simulink model "SIFT_final"  (R2015a)
settings: Solver=ode45  StartTime=0.0  StopTime=10.0  RelTol=1e-3
InitFcn:
  | %% DSPBuilder Start
  | alt_dspbuilder_update_model(bdroot)
  | %% DSPBuilder End
libraries: allblocks_alteradspbuilder2 x1826
(part 2 of 24)

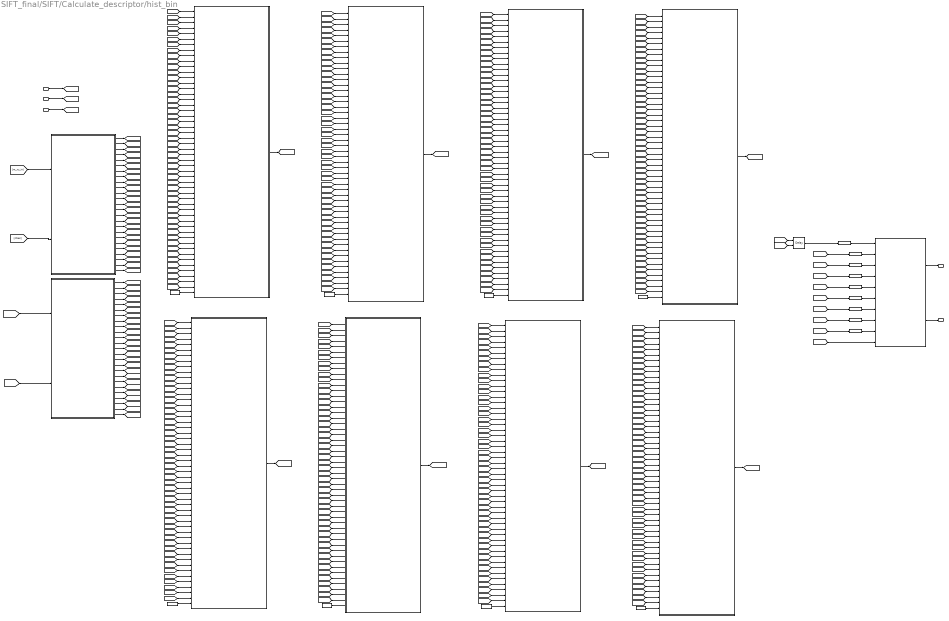
== system SIFT_final/SIFT/Calculate_descriptor/hist_bin ==
  m_xy_In : Inport
  orien_In : Inport  Port=2
  clken : Inport  Port=3
  AltBus : allblocks_alteradspbuilder2/AltBus  BusType=Unsigned Integer  bwl=16  bwr=0  saturate=off  floatingPointInput=on  floatingPointOutput=on  logOutputs=off  logFile=C:\Users\ASUS\Desktop\final_sift_fpga\tb_SIFT_final\SIFT%5Ffinal_SIFT_Calculate%5Fdescriptor_hist%5Fbin_AltBus.fixedpointlog
  AltBus1 : allblocks_alteradspbuilder2/AltBus  BusType=Unsigned Integer  bwl=16  bwr=0  saturate=off  floatingPointInput=on  floatingPointOutput=on  logOutputs=off  logFile=C:\Users\ASUS\Desktop\final_sift_fpga\tb_SIFT_final\SIFT%5Ffinal_SIFT_Calculate%5Fdescriptor_hist%5Fbin_AltBus1.fixedpointlog
  AltBus2 : allblocks_alteradspbuilder2/AltBus  BusType=Unsigned Integer  bwl=16  bwr=0  saturate=off  floatingPointInput=on  floatingPointOutput=on  logOutputs=off  logFile=C:\Users\ASUS\Desktop\final_sift_fpga\tb_SIFT_final\SIFT%5Ffinal_SIFT_Calculate%5Fdescriptor_hist%5Fbin_AltBus2.fixedpointlog
  AltBus3 : allblocks_alteradspbuilder2/AltBus  BusType=Unsigned Integer  bwl=16  bwr=0  saturate=off  floatingPointInput=on  floatingPointOutput=on  logOutputs=off  logFile=C:\Users\ASUS\Desktop\final_sift_fpga\tb_SIFT_final\SIFT%5Ffinal_SIFT_Calculate%5Fdescriptor_hist%5Fbin_AltBus3.fixedpointlog
  AltBus4 : allblocks_alteradspbuilder2/AltBus  BusType=Unsigned Integer  bwl=16  bwr=0  saturate=off  floatingPointInput=on  floatingPointOutput=on  logOutputs=off  logFile=C:\Users\ASUS\Desktop\final_sift_fpga\tb_SIFT_final\SIFT%5Ffinal_SIFT_Calculate%5Fdescriptor_hist%5Fbin_AltBus4.fixedpointlog
  AltBus5 : allblocks_alteradspbuilder2/AltBus  BusType=Unsigned Integer  bwl=16  bwr=0  saturate=off  floatingPointInput=on  floatingPointOutput=on  logOutputs=off  logFile=C:\Users\ASUS\Desktop\final_sift_fpga\tb_SIFT_final\SIFT%5Ffinal_SIFT_Calculate%5Fdescriptor_hist%5Fbin_AltBus5.fixedpointlog
  AltBus6 : allblocks_alteradspbuilder2/AltBus  BusType=Unsigned Integer  bwl=16  bwr=0  saturate=off  floatingPointInput=on  floatingPointOutput=on  logOutputs=off  logFile=C:\Users\ASUS\Desktop\final_sift_fpga\tb_SIFT_final\SIFT%5Ffinal_SIFT_Calculate%5Fdescriptor_hist%5Fbin_AltBus6.fixedpointlog
  AltBus7 : allblocks_alteradspbuilder2/AltBus  BusType=Unsigned Integer  bwl=16  bwr=0  saturate=off  floatingPointInput=on  floatingPointOutput=on  logOutputs=off  logFile=C:\Users\ASUS\Desktop\final_sift_fpga\tb_SIFT_final\SIFT%5Ffinal_SIFT_Calculate%5Fdescriptor_hist%5Fbin_AltBus7.fixedpointlog
  AltBus8 : allblocks_alteradspbuilder2/AltBus  BusType=Unsigned Integer  bwl=3  bwr=0  saturate=off  floatingPointInput=on  floatingPointOutput=on  logOutputs=off  logFile=C:\Users\ASUS\Desktop\final_sift_fpga\tb_SIFT_final\SIFT%5Ffinal_SIFT_Calculate%5Fdescriptor_hist%5Fbin_AltBus8.fixedpointlog
  Bus_Concatenation : Subsystem
  Constant : allblocks_alteradspbuilder2/Constant  mask_cst=0  BusType=Unsigned Integer  bwl=8  bwr=0  roundMode=Truncate  satMode=Wrap  SpecifyClock=off  allowFloatingPointOverride=on  logOutputs=off  logFile=C:\Users\ASUS\Desktop\final_sift_fpga\tb_SIFT_final\SIFT%5Ffinal_SIFT_Calculate%5Fdescriptor_hist%5Fbin_Constant.fixedpointlog
  Constant1 : allblocks_alteradspbuilder2/Constant  mask_cst=1  BusType=Unsigned Integer  bwl=8  bwr=0  roundMode=Truncate  satMode=Wrap  SpecifyClock=off  allowFloatingPointOverride=on  logOutputs=off  logFile=C:\Users\ASUS\Desktop\final_sift_fpga\tb_SIFT_final\SIFT%5Ffinal_SIFT_Calculate%5Fdescriptor_hist%5Fbin_Constant1.fixedpointlog
  Constant2 : allblocks_alteradspbuilder2/Constant  mask_cst=2  BusType=Unsigned Integer  bwl=8  bwr=0  roundMode=Truncate  satMode=Wrap  SpecifyClock=off  allowFloatingPointOverride=on  logOutputs=off  logFile=C:\Users\ASUS\Desktop\final_sift_fpga\tb_SIFT_final\SIFT%5Ffinal_SIFT_Calculate%5Fdescriptor_hist%5Fbin_Constant2.fixedpointlog
  Constant3 : allblocks_alteradspbuilder2/Constant  mask_cst=3  BusType=Unsigned Integer  bwl=8  bwr=0  roundMode=Truncate  satMode=Wrap  SpecifyClock=off  allowFloatingPointOverride=on  logOutputs=off  logFile=C:\Users\ASUS\Desktop\final_sift_fpga\tb_SIFT_final\SIFT%5Ffinal_SIFT_Calculate%5Fdescriptor_hist%5Fbin_Constant3.fixedpointlog
  Constant4 : allblocks_alteradspbuilder2/Constant  mask_cst=4  BusType=Unsigned Integer  bwl=8  bwr=0  roundMode=Truncate  satMode=Wrap  SpecifyClock=off  allowFloatingPointOverride=on  logOutputs=off  logFile=C:\Users\ASUS\Desktop\final_sift_fpga\tb_SIFT_final\SIFT%5Ffinal_SIFT_Calculate%5Fdescriptor_hist%5Fbin_Constant4.fixedpointlog
  Constant5 : allblocks_alteradspbuilder2/Constant  mask_cst=5  BusType=Unsigned Integer  bwl=8  bwr=0  roundMode=Truncate  satMode=Wrap  SpecifyClock=off  allowFloatingPointOverride=on  logOutputs=off  logFile=C:\Users\ASUS\Desktop\final_sift_fpga\tb_SIFT_final\SIFT%5Ffinal_SIFT_Calculate%5Fdescriptor_hist%5Fbin_Constant5.fixedpointlog
  Constant6 : allblocks_alteradspbuilder2/Constant  mask_cst=6  BusType=Unsigned Integer  bwl=8  bwr=0  roundMode=Truncate  satMode=Wrap  SpecifyClock=off  allowFloatingPointOverride=on  logOutputs=off  logFile=C:\Users\ASUS\Desktop\final_sift_fpga\tb_SIFT_final\SIFT%5Ffinal_SIFT_Calculate%5Fdescriptor_hist%5Fbin_Constant6.fixedpointlog
  Constant7 : allblocks_alteradspbuilder2/Constant  mask_cst=7  BusType=Unsigned Integer  bwl=8  bwr=0  roundMode=Truncate  satMode=Wrap  SpecifyClock=off  allowFloatingPointOverride=on  logOutputs=off  logFile=C:\Users\ASUS\Desktop\final_sift_fpga\tb_SIFT_final\SIFT%5Ffinal_SIFT_Calculate%5Fdescriptor_hist%5Fbin_Constant7.fixedpointlog
  Delay : allblocks_alteradspbuilder2/Delay  pipeline=5+16  pipeline_display=21  ClockPhase=1  use_ena=on  use_sclr=off  allowFloatingPointOverride=on  logOutputs=off  logFile=C:\Users\ASUS\Desktop\final_sift_fpga\tb_SIFT_final\SIFT%5Ffinal_SIFT_Calculate%5Fdescriptor_hist%5Fbin_Delay.fixedpointlog  use_init=off  reset_value=1
  Line_buffer_5x5 : Subsystem
  Line_buffer_5x5_1 : Subsystem
  hist_bin1 : Subsystem
  hist_bin2 : Subsystem
  hist_bin3 : Subsystem
  hist_bin4 : Subsystem
  hist_bin5 : Subsystem
  hist_bin6 : Subsystem
  hist_bin7 : Subsystem
  hist_bin8 : Subsystem
  hist_bin_out : Outport
  Orien_out : Outport  Port=2
  wires:
  [m_xy_in] -> Line_buffer_5x5/1(dataIn)
  [clken] -> Line_buffer_5x5/2(clken)
  [clken] -> Line_buffer_5x5_1/2(clken)
  [orien_in] -> Line_buffer_5x5_1/1(dataIn)
  clken/1 -> [clken]
  Line_buffer_5x5_1/21(Out40) -> [orien_40]
  Line_buffer_5x5_1/19(Out33) -> [orien_33]
  Line_buffer_5x5_1/8(Out12) -> [orien_12]
  Line_buffer_5x5_1/14(Out23) -> [orien_23]
  Line_buffer_5x5_1/18(Out32) -> [orien_32]
  Line_buffer_5x5_1/20(Out34) -> [orien_34]
  Line_buffer_5x5_1/2(Out01) -> [orien_01]
  Line_buffer_5x5_1/7(Out11) -> [orien_11]
  Line_buffer_5x5_1/11(Out20) -> [orien_20]
  Line_buffer_5x5_1/13(Out22) -> [orien_22]
  Line_buffer_5x5_1/17(Out31) -> [orien_31]
  Line_buffer_5x5_1/25(Out44) -> [orien_44]
  Line_buffer_5x5_1/3(Out02) -> [orien_02]
  Line_buffer_5x5_1/5(Out04) -> [orien_04]
  Line_buffer_5x5_1/23(Out42) -> [orien_42]
  Line_buffer_5x5_1/24(Out43) -> [orien_43]
  Line_buffer_5x5_1/6(Out10) -> [orien_10]
  Line_buffer_5x5_1/1(Out00) -> [orien_00]
  Line_buffer_5x5_1/22(Out41) -> [orien_41]
  Line_buffer_5x5_1/15(Out24) -> [orien_24]
  Line_buffer_5x5_1/4(Out03) -> [orien_03]
  Line_buffer_5x5_1/9(Out13) -> [orien_13]
  Line_buffer_5x5_1/10(Out14) -> [orien_14]
  Line_buffer_5x5_1/12(Out21) -> [orien_21]
  Line_buffer_5x5_1/16(Out30) -> [orien_30]
  Line_buffer_5x5/24(Out43) -> [m_xy_43]
  Line_buffer_5x5/21(Out40) -> [m_xy_40]
  Line_buffer_5x5/23(Out42) -> [m_xy_42]
  Line_buffer_5x5/22(Out41) -> [m_xy_41]
  Line_buffer_5x5/25(Out44) -> [m_xy_44]
  Line_buffer_5x5/12(Out21) -> [m_xy_21]
  Line_buffer_5x5/15(Out24) -> [m_xy_24]
  Line_buffer_5x5/19(Out33) -> [m_xy_33]
  Line_buffer_5x5/18(Out32) -> [m_xy_32]
  Line_buffer_5x5/13(Out22) -> [m_xy_22]
  Line_buffer_5x5/11(Out20) -> [m_xy_20]
  Line_buffer_5x5/16(Out30) -> [m_xy_30]
  Line_buffer_5x5/14(Out23) -> [m_xy_23]
  Line_buffer_5x5/17(Out31) -> [m_xy_31]
  Line_buffer_5x5/20(Out34) -> [m_xy_34]
  Line_buffer_5x5/1(Out00) -> [m_xy_00]
  [m_xy_04] -> hist_bin1/5(Mxy_In04)
  Line_buffer_5x5/2(Out01) -> [m_xy_01]
  hist_bin1/1(bin_out) -> [hist_bin1]
  [m_xy_10] -> hist_bin1/6(Mxy_In10)
  Line_buffer_5x5/9(Out13) -> [m_xy_13]
  [m_xy_13] -> hist_bin1/9(Mxy_In13)
  Line_buffer_5x5/10(Out14) -> [m_xy_14]
  Line_buffer_5x5/6(Out10) -> [m_xy_10]
  Line_buffer_5x5/7(Out11) -> [m_xy_11]
  [m_xy_11] -> hist_bin1/7(Mxy_In11)
  [m_xy_12] -> hist_bin1/8(Mxy_In12)
  Line_buffer_5x5/8(Out12) -> [m_xy_12]
  [m_xy_14] -> hist_bin1/10(Mxy_In14)
  [m_xy_22] -> hist_bin1/13(Mxy_In22)
  [m_xy_40] -> hist_bin1/21(Mxy_In40)
  [m_xy_43] -> hist_bin1/24(Mxy_In43)
  [m_xy_42] -> hist_bin1/23(Mxy_In42)
  [m_xy_44] -> hist_bin1/25(Mxy_In44)
  [m_xy_24] -> hist_bin1/15(Mxy_In24)
  [m_xy_21] -> hist_bin1/12(Mxy_In21)
  [m_xy_20] -> hist_bin1/11(Mxy_In20)
  [m_xy_23] -> hist_bin1/14(Mxy_In23)
  [m_xy_41] -> hist_bin1/22(Mxy_In41)
  [m_xy_01] -> hist_bin1/2(Mxy_In01)
  Line_buffer_5x5/4(Out03) -> [m_xy_03]
  Line_buffer_5x5/5(Out04) -> [m_xy_04]
  Line_buffer_5x5/3(Out02) -> [m_xy_02]
  [m_xy_31] -> hist_bin1/17(Mxy_In31)
  [m_xy_30] -> hist_bin1/16(Mxy_In30)
  [m_xy_34] -> hist_bin1/20(Mxy_In34)
  [m_xy_33] -> hist_bin1/19(Mxy_In33)
  [m_xy_32] -> hist_bin1/18(Mxy_In32)
  [m_xy_03] -> hist_bin1/4(Mxy_In03)
  [m_xy_02] -> hist_bin1/3(Mxy_In02)
  [orien_10] -> hist_bin1/31(Orien_In10)
  [orien_42] -> hist_bin1/48(Orien_In42)
  [orien_01] -> hist_bin1/27(Orien_In01)
  [orien_20] -> hist_bin1/36(Orien_In20)
  [orien_31] -> hist_bin1/42(Orien_In31)
  [orien_33] -> hist_bin1/44(Orien_In33)
  [orien_21] -> hist_bin1/37(Orien_In21)
  [orien_24] -> hist_bin1/40(Orien_In24)
  [orien_03] -> hist_bin1/29(Orien_In03)
  [orien_30] -> hist_bin1/41(Orien_In30)
  [orien_12] -> hist_bin1/33(Orien_In12)
  [orien_23] -> hist_bin1/39(Orien_In23)
  [orien_32] -> hist_bin1/43(Orien_In32)
  [orien_41] -> hist_bin1/47(Orien_In41)
  [orien_43] -> hist_bin1/49(Orien_In43)
  [orien_02] -> hist_bin1/28(Orien_In02)
  [orien_00] -> hist_bin1/26(Orien_In00)
  [orien_11] -> hist_bin1/32(Orien_In11)
  [orien_34] -> hist_bin1/45(Orien_In34)
  [orien_22] -> hist_bin1/38(Orien_In22)
  [orien_04] -> hist_bin1/30(Orien_In04)
  [orien_14] -> hist_bin1/35(Orien_In14)
  [orien_44] -> hist_bin1/50(Orien_In44)
  [orien_13] -> hist_bin1/34(Orien_In13)
  [orien_40] -> hist_bin1/46(Orien_In40)
  [clken] -> hist_bin1/51(clken)
  Constant/1 -> hist_bin1/52(bin_in)
  [m_xy_02] -> hist_bin2/3(Mxy_In02)
  [m_xy_04] -> hist_bin2/5(Mxy_In04)
  [m_xy_10] -> hist_bin2/6(Mxy_In10)
  [m_xy_23] -> hist_bin2/14(Mxy_In23)
  [m_xy_31] -> hist_bin2/17(Mxy_In31)
  [m_xy_30] -> hist_bin2/16(Mxy_In30)
  [m_xy_12] -> hist_bin2/8(Mxy_In12)
  [m_xy_32] -> hist_bin2/18(Mxy_In32)
  [m_xy_13] -> hist_bin2/9(Mxy_In13)
  [m_xy_33] -> hist_bin2/19(Mxy_In33)
  [m_xy_41] -> hist_bin2/22(Mxy_In41)
  [m_xy_01] -> hist_bin2/2(Mxy_In01)
  [m_xy_14] -> hist_bin2/10(Mxy_In14)
  [m_xy_40] -> hist_bin2/21(Mxy_In40)
  [m_xy_43] -> hist_bin2/24(Mxy_In43)
  [m_xy_20] -> hist_bin2/11(Mxy_In20)
  [m_xy_22] -> hist_bin2/13(Mxy_In22)
  [m_xy_24] -> hist_bin2/15(Mxy_In24)
  [m_xy_34] -> hist_bin2/20(Mxy_In34)
  [m_xy_03] -> hist_bin2/4(Mxy_In03)
  [m_xy_00] -> hist_bin2/1(Mxy_In00)
  [m_xy_11] -> hist_bin2/7(Mxy_In11)
  [m_xy_21] -> hist_bin2/12(Mxy_In21)
  [orien_31] -> hist_bin2/42(Orien_In31)
  [orien_34] -> hist_bin2/45(Orien_In34)
  [m_xy_42] -> hist_bin2/23(Mxy_In42)
  [orien_01] -> hist_bin2/27(Orien_In01)
  [orien_00] -> hist_bin2/26(Orien_In00)
  [orien_04] -> hist_bin2/30(Orien_In04)
  [orien_13] -> hist_bin2/34(Orien_In13)
  [orien_20] -> hist_bin2/36(Orien_In20)
  [orien_24] -> hist_bin2/40(Orien_In24)
  [orien_33] -> hist_bin2/44(Orien_In33)
  [orien_32] -> hist_bin2/43(Orien_In32)
  [orien_41] -> hist_bin2/47(Orien_In41)
  [orien_11] -> hist_bin2/32(Orien_In11)
  [orien_21] -> hist_bin2/37(Orien_In21)
  [orien_14] -> hist_bin2/35(Orien_In14)
  [orien_22] -> hist_bin2/38(Orien_In22)
  [orien_23] -> hist_bin2/39(Orien_In23)
  [orien_02] -> hist_bin2/28(Orien_In02)
  [orien_10] -> hist_bin2/31(Orien_In10)
  [orien_12] -> hist_bin2/33(Orien_In12)
  [orien_30] -> hist_bin2/41(Orien_In30)
  [m_xy_44] -> hist_bin2/25(Mxy_In44)
  [orien_03] -> hist_bin2/29(Orien_In03)
  [orien_40] -> hist_bin2/46(Orien_In40)
  [clken] -> hist_bin2/51(clken)
  hist_bin2/1(bin_out) -> [hist_bin2]
  [orien_42] -> hist_bin2/48(Orien_In42)
  [orien_44] -> hist_bin2/50(Orien_In44)
  [orien_43] -> hist_bin2/49(Orien_In43)
  Constant1/1 -> hist_bin2/52(bin_in)
  [m_xy_00] -> hist_bin1/1(Mxy_In00)
  orien_In/1 -> [orien_in]
  m_xy_In/1 -> [m_xy_in]
  [m_xy_04] -> hist_bin3/5(Mxy_In04)
  hist_bin3/1(bin_out) -> [hist_bin3]
  [m_xy_10] -> hist_bin3/6(Mxy_In10)
  [m_xy_13] -> hist_bin3/9(Mxy_In13)
  [m_xy_11] -> hist_bin3/7(Mxy_In11)
  [m_xy_12] -> hist_bin3/8(Mxy_In12)
  [m_xy_14] -> hist_bin3/10(Mxy_In14)
  [m_xy_22] -> hist_bin3/13(Mxy_In22)
  [m_xy_40] -> hist_bin3/21(Mxy_In40)
  [m_xy_43] -> hist_bin3/24(Mxy_In43)
  [m_xy_42] -> hist_bin3/23(Mxy_In42)
  [m_xy_44] -> hist_bin3/25(Mxy_In44)
  [m_xy_24] -> hist_bin3/15(Mxy_In24)
  [m_xy_21] -> hist_bin3/12(Mxy_In21)
  [m_xy_20] -> hist_bin3/11(Mxy_In20)
  [m_xy_23] -> hist_bin3/14(Mxy_In23)
  [m_xy_41] -> hist_bin3/22(Mxy_In41)
  [m_xy_01] -> hist_bin3/2(Mxy_In01)
  [m_xy_31] -> hist_bin3/17(Mxy_In31)
  [m_xy_30] -> hist_bin3/16(Mxy_In30)
  [m_xy_34] -> hist_bin3/20(Mxy_In34)
  [m_xy_33] -> hist_bin3/19(Mxy_In33)
  [m_xy_32] -> hist_bin3/18(Mxy_In32)
  [m_xy_03] -> hist_bin3/4(Mxy_In03)
  [m_xy_02] -> hist_bin3/3(Mxy_In02)
  [orien_10] -> hist_bin3/31(Orien_In10)
  [orien_42] -> hist_bin3/48(Orien_In42)
  [orien_01] -> hist_bin3/27(Orien_In01)
  [orien_20] -> hist_bin3/36(Orien_In20)
  [orien_31] -> hist_bin3/42(Orien_In31)
  [orien_33] -> hist_bin3/44(Orien_In33)
  [orien_21] -> hist_bin3/37(Orien_In21)
  [orien_24] -> hist_bin3/40(Orien_In24)
  [orien_03] -> hist_bin3/29(Orien_In03)
  [orien_30] -> hist_bin3/41(Orien_In30)
  [orien_12] -> hist_bin3/33(Orien_In12)
  [orien_23] -> hist_bin3/39(Orien_In23)
  [orien_32] -> hist_bin3/43(Orien_In32)
  [orien_41] -> hist_bin3/47(Orien_In41)
  [orien_43] -> hist_bin3/49(Orien_In43)
  [orien_02] -> hist_bin3/28(Orien_In02)
  [orien_00] -> hist_bin3/26(Orien_In00)
  [orien_11] -> hist_bin3/32(Orien_In11)
  [orien_34] -> hist_bin3/45(Orien_In34)
  [orien_22] -> hist_bin3/38(Orien_In22)
  [orien_04] -> hist_bin3/30(Orien_In04)
  [orien_14] -> hist_bin3/35(Orien_In14)
  [orien_44] -> hist_bin3/50(Orien_In44)
  [orien_13] -> hist_bin3/34(Orien_In13)
  [orien_40] -> hist_bin3/46(Orien_In40)
  [clken] -> hist_bin3/51(clken)
  Constant2/1 -> hist_bin3/52(bin_in)
  [m_xy_02] -> hist_bin4/3(Mxy_In02)
  [m_xy_04] -> hist_bin4/5(Mxy_In04)
  [m_xy_10] -> hist_bin4/6(Mxy_In10)
  [m_xy_23] -> hist_bin4/14(Mxy_In23)
  [m_xy_31] -> hist_bin4/17(Mxy_In31)
  [m_xy_30] -> hist_bin4/16(Mxy_In30)
  [m_xy_12] -> hist_bin4/8(Mxy_In12)
  [m_xy_32] -> hist_bin4/18(Mxy_In32)
  [m_xy_13] -> hist_bin4/9(Mxy_In13)
  [m_xy_33] -> hist_bin4/19(Mxy_In33)
  [m_xy_41] -> hist_bin4/22(Mxy_In41)
  [m_xy_01] -> hist_bin4/2(Mxy_In01)
  [m_xy_14] -> hist_bin4/10(Mxy_In14)
  [m_xy_40] -> hist_bin4/21(Mxy_In40)
  [m_xy_43] -> hist_bin4/24(Mxy_In43)
  [m_xy_20] -> hist_bin4/11(Mxy_In20)
  [m_xy_22] -> hist_bin4/13(Mxy_In22)
  [m_xy_24] -> hist_bin4/15(Mxy_In24)
  [m_xy_34] -> hist_bin4/20(Mxy_In34)
  [m_xy_03] -> hist_bin4/4(Mxy_In03)
  [m_xy_00] -> hist_bin4/1(Mxy_In00)
  [m_xy_11] -> hist_bin4/7(Mxy_In11)
  [m_xy_21] -> hist_bin4/12(Mxy_In21)
  [orien_31] -> hist_bin4/42(Orien_In31)
  [orien_34] -> hist_bin4/45(Orien_In34)
  [m_xy_42] -> hist_bin4/23(Mxy_In42)
  [orien_01] -> hist_bin4/27(Orien_In01)
  [orien_00] -> hist_bin4/26(Orien_In00)
  [orien_04] -> hist_bin4/30(Orien_In04)
  [orien_13] -> hist_bin4/34(Orien_In13)
  [orien_20] -> hist_bin4/36(Orien_In20)
  [orien_24] -> hist_bin4/40(Orien_In24)
  [orien_33] -> hist_bin4/44(Orien_In33)
  [orien_32] -> hist_bin4/43(Orien_In32)
  [orien_41] -> hist_bin4/47(Orien_In41)
  [orien_11] -> hist_bin4/32(Orien_In11)
  [orien_21] -> hist_bin4/37(Orien_In21)
  [orien_14] -> hist_bin4/35(Orien_In14)
  [orien_22] -> hist_bin4/38(Orien_In22)
  [orien_23] -> hist_bin4/39(Orien_In23)
  [orien_02] -> hist_bin4/28(Orien_In02)
  [orien_10] -> hist_bin4/31(Orien_In10)
  [orien_12] -> hist_bin4/33(Orien_In12)
  [orien_30] -> hist_bin4/41(Orien_In30)
  [m_xy_44] -> hist_bin4/25(Mxy_In44)
  [orien_03] -> hist_bin4/29(Orien_In03)
  [orien_40] -> hist_bin4/46(Orien_In40)
  [clken] -> hist_bin4/51(clken)
  hist_bin4/1(bin_out) -> [hist_bin4]
  [orien_42] -> hist_bin4/48(Orien_In42)
  [orien_44] -> hist_bin4/50(Orien_In44)
  [orien_43] -> hist_bin4/49(Orien_In43)
  Constant3/1 -> hist_bin4/52(bin_in)
  [m_xy_00] -> hist_bin3/1(Mxy_In00)
  [m_xy_04] -> hist_bin5/5(Mxy_In04)
  hist_bin5/1(bin_out) -> [hist_bin5]
  [m_xy_10] -> hist_bin5/6(Mxy_In10)
  [m_xy_13] -> hist_bin5/9(Mxy_In13)
  [m_xy_11] -> hist_bin5/7(Mxy_In11)
  [m_xy_12] -> hist_bin5/8(Mxy_In12)
  [m_xy_14] -> hist_bin5/10(Mxy_In14)
  [m_xy_22] -> hist_bin5/13(Mxy_In22)
  [m_xy_40] -> hist_bin5/21(Mxy_In40)
  [m_xy_43] -> hist_bin5/24(Mxy_In43)
  [m_xy_42] -> hist_bin5/23(Mxy_In42)
  [m_xy_44] -> hist_bin5/25(Mxy_In44)
  [m_xy_24] -> hist_bin5/15(Mxy_In24)
  [m_xy_21] -> hist_bin5/12(Mxy_In21)
  [m_xy_20] -> hist_bin5/11(Mxy_In20)
  [m_xy_23] -> hist_bin5/14(Mxy_In23)
  [m_xy_41] -> hist_bin5/22(Mxy_In41)
  [m_xy_01] -> hist_bin5/2(Mxy_In01)
  [m_xy_31] -> hist_bin5/17(Mxy_In31)
  [m_xy_30] -> hist_bin5/16(Mxy_In30)
  [m_xy_34] -> hist_bin5/20(Mxy_In34)
  [m_xy_33] -> hist_bin5/19(Mxy_In33)
  [m_xy_32] -> hist_bin5/18(Mxy_In32)
  [m_xy_03] -> hist_bin5/4(Mxy_In03)
  [m_xy_02] -> hist_bin5/3(Mxy_In02)
  [orien_10] -> hist_bin5/31(Orien_In10)
  [orien_42] -> hist_bin5/48(Orien_In42)
  [orien_01] -> hist_bin5/27(Orien_In01)
  [orien_20] -> hist_bin5/36(Orien_In20)
  [orien_31] -> hist_bin5/42(Orien_In31)
  [orien_33] -> hist_bin5/44(Orien_In33)
  [orien_21] -> hist_bin5/37(Orien_In21)
  [orien_24] -> hist_bin5/40(Orien_In24)
  [orien_03] -> hist_bin5/29(Orien_In03)
  [orien_30] -> hist_bin5/41(Orien_In30)
  [orien_12] -> hist_bin5/33(Orien_In12)
  [orien_23] -> hist_bin5/39(Orien_In23)
  [orien_32] -> hist_bin5/43(Orien_In32)
  [orien_41] -> hist_bin5/47(Orien_In41)
  [orien_43] -> hist_bin5/49(Orien_In43)
  [orien_02] -> hist_bin5/28(Orien_In02)
  [orien_00] -> hist_bin5/26(Orien_In00)
  [orien_11] -> hist_bin5/32(Orien_In11)
  [orien_34] -> hist_bin5/45(Orien_In34)
  [orien_22] -> hist_bin5/38(Orien_In22)
  [orien_04] -> hist_bin5/30(Orien_In04)
  [orien_14] -> hist_bin5/35(Orien_In14)
  [orien_44] -> hist_bin5/50(Orien_In44)
  [orien_13] -> hist_bin5/34(Orien_In13)
  [orien_40] -> hist_bin5/46(Orien_In40)
  [clken] -> hist_bin5/51(clken)
  Constant4/1 -> hist_bin5/52(bin_in)
  [m_xy_02] -> hist_bin6/3(Mxy_In02)
  [m_xy_04] -> hist_bin6/5(Mxy_In04)
  [m_xy_10] -> hist_bin6/6(Mxy_In10)
  [m_xy_23] -> hist_bin6/14(Mxy_In23)
  [m_xy_31] -> hist_bin6/17(Mxy_In31)
  [m_xy_30] -> hist_bin6/16(Mxy_In30)
  [m_xy_12] -> hist_bin6/8(Mxy_In12)
  [m_xy_32] -> hist_bin6/18(Mxy_In32)
  [m_xy_13] -> hist_bin6/9(Mxy_In13)
  [m_xy_33] -> hist_bin6/19(Mxy_In33)
  [m_xy_41] -> hist_bin6/22(Mxy_In41)
  [m_xy_01] -> hist_bin6/2(Mxy_In01)
  [m_xy_14] -> hist_bin6/10(Mxy_In14)
  [m_xy_40] -> hist_bin6/21(Mxy_In40)
  [m_xy_43] -> hist_bin6/24(Mxy_In43)
  [m_xy_20] -> hist_bin6/11(Mxy_In20)
  [m_xy_22] -> hist_bin6/13(Mxy_In22)
  [m_xy_24] -> hist_bin6/15(Mxy_In24)
  [m_xy_34] -> hist_bin6/20(Mxy_In34)
  [m_xy_03] -> hist_bin6/4(Mxy_In03)
  [m_xy_00] -> hist_bin6/1(Mxy_In00)
  [m_xy_11] -> hist_bin6/7(Mxy_In11)
  [m_xy_21] -> hist_bin6/12(Mxy_In21)
  [orien_31] -> hist_bin6/42(Orien_In31)
  [orien_34] -> hist_bin6/45(Orien_In34)
  [m_xy_42] -> hist_bin6/23(Mxy_In42)
  [orien_01] -> hist_bin6/27(Orien_In01)
  [orien_00] -> hist_bin6/26(Orien_In00)
  [orien_04] -> hist_bin6/30(Orien_In04)
  [orien_13] -> hist_bin6/34(Orien_In13)
  [orien_20] -> hist_bin6/36(Orien_In20)
  [orien_24] -> hist_bin6/40(Orien_In24)
  [orien_33] -> hist_bin6/44(Orien_In33)
  [orien_32] -> hist_bin6/43(Orien_In32)
  [orien_41] -> hist_bin6/47(Orien_In41)
  [orien_11] -> hist_bin6/32(Orien_In11)
  [orien_21] -> hist_bin6/37(Orien_In21)
  [orien_14] -> hist_bin6/35(Orien_In14)
  [orien_22] -> hist_bin6/38(Orien_In22)
  [orien_23] -> hist_bin6/39(Orien_In23)
  [orien_02] -> hist_bin6/28(Orien_In02)
  [orien_10] -> hist_bin6/31(Orien_In10)
  [orien_12] -> hist_bin6/33(Orien_In12)
  [orien_30] -> hist_bin6/41(Orien_In30)
  [m_xy_44] -> hist_bin6/25(Mxy_In44)
  [orien_03] -> hist_bin6/29(Orien_In03)
  [orien_40] -> hist_bin6/46(Orien_In40)
  [clken] -> hist_bin6/51(clken)
  hist_bin6/1(bin_out) -> [hist_bin6]
  [orien_42] -> hist_bin6/48(Orien_In42)
  [orien_44] -> hist_bin6/50(Orien_In44)
  [orien_43] -> hist_bin6/49(Orien_In43)
  Constant5/1 -> hist_bin6/52(bin_in)
  [m_xy_00] -> hist_bin5/1(Mxy_In00)
  [m_xy_04] -> hist_bin7/5(Mxy_In04)
  hist_bin7/1(bin_out) -> [hist_bin7]
  [m_xy_10] -> hist_bin7/6(Mxy_In10)
  [m_xy_13] -> hist_bin7/9(Mxy_In13)
  [m_xy_11] -> hist_bin7/7(Mxy_In11)
  [m_xy_12] -> hist_bin7/8(Mxy_In12)
  [m_xy_14] -> hist_bin7/10(Mxy_In14)
  [m_xy_22] -> hist_bin7/13(Mxy_In22)
  [m_xy_40] -> hist_bin7/21(Mxy_In40)
  [m_xy_43] -> hist_bin7/24(Mxy_In43)
  [m_xy_42] -> hist_bin7/23(Mxy_In42)
  [m_xy_44] -> hist_bin7/25(Mxy_In44)
  [m_xy_24] -> hist_bin7/15(Mxy_In24)
  [m_xy_21] -> hist_bin7/12(Mxy_In21)
  [m_xy_20] -> hist_bin7/11(Mxy_In20)
  [m_xy_23] -> hist_bin7/14(Mxy_In23)
  [m_xy_41] -> hist_bin7/22(Mxy_In41)
  [m_xy_01] -> hist_bin7/2(Mxy_In01)
  [m_xy_31] -> hist_bin7/17(Mxy_In31)
  [m_xy_30] -> hist_bin7/16(Mxy_In30)
  [m_xy_34] -> hist_bin7/20(Mxy_In34)
  [m_xy_33] -> hist_bin7/19(Mxy_In33)
  [m_xy_32] -> hist_bin7/18(Mxy_In32)
  [m_xy_03] -> hist_bin7/4(Mxy_In03)
  [m_xy_02] -> hist_bin7/3(Mxy_In02)
  [orien_10] -> hist_bin7/31(Orien_In10)
  [orien_42] -> hist_bin7/48(Orien_In42)
  [orien_01] -> hist_bin7/27(Orien_In01)
  [orien_20] -> hist_bin7/36(Orien_In20)
  [orien_31] -> hist_bin7/42(Orien_In31)
  [orien_33] -> hist_bin7/44(Orien_In33)
  [orien_21] -> hist_bin7/37(Orien_In21)
  [orien_24] -> hist_bin7/40(Orien_In24)
  [orien_03] -> hist_bin7/29(Orien_In03)
  [orien_30] -> hist_bin7/41(Orien_In30)
  [orien_12] -> hist_bin7/33(Orien_In12)
  [orien_23] -> hist_bin7/39(Orien_In23)
  [orien_32] -> hist_bin7/43(Orien_In32)
  [orien_41] -> hist_bin7/47(Orien_In41)
  [orien_43] -> hist_bin7/49(Orien_In43)
  [orien_02] -> hist_bin7/28(Orien_In02)
  [orien_00] -> hist_bin7/26(Orien_In00)
  [orien_11] -> hist_bin7/32(Orien_In11)
  [orien_34] -> hist_bin7/45(Orien_In34)
  [orien_22] -> hist_bin7/38(Orien_In22)
  [orien_04] -> hist_bin7/30(Orien_In04)
  [orien_14] -> hist_bin7/35(Orien_In14)
  [orien_44] -> hist_bin7/50(Orien_In44)
  [orien_13] -> hist_bin7/34(Orien_In13)
  [orien_40] -> hist_bin7/46(Orien_In40)
  [clken] -> hist_bin7/51(clken)
  Constant6/1 -> hist_bin7/52(bin_in)
  [m_xy_02] -> hist_bin8/3(Mxy_In02)
  [m_xy_04] -> hist_bin8/5(Mxy_In04)
  [m_xy_10] -> hist_bin8/6(Mxy_In10)
  [m_xy_23] -> hist_bin8/14(Mxy_In23)
  [m_xy_31] -> hist_bin8/17(Mxy_In31)
  [m_xy_30] -> hist_bin8/16(Mxy_In30)
  [m_xy_12] -> hist_bin8/8(Mxy_In12)
  [m_xy_32] -> hist_bin8/18(Mxy_In32)
  [m_xy_13] -> hist_bin8/9(Mxy_In13)
  [m_xy_33] -> hist_bin8/19(Mxy_In33)
  [m_xy_41] -> hist_bin8/22(Mxy_In41)
  [m_xy_01] -> hist_bin8/2(Mxy_In01)
  [m_xy_14] -> hist_bin8/10(Mxy_In14)
  [m_xy_40] -> hist_bin8/21(Mxy_In40)
  [m_xy_43] -> hist_bin8/24(Mxy_In43)
  [m_xy_20] -> hist_bin8/11(Mxy_In20)
  [m_xy_22] -> hist_bin8/13(Mxy_In22)
  [m_xy_24] -> hist_bin8/15(Mxy_In24)
  [m_xy_34] -> hist_bin8/20(Mxy_In34)
  [m_xy_03] -> hist_bin8/4(Mxy_In03)
  [m_xy_00] -> hist_bin8/1(Mxy_In00)
  [m_xy_11] -> hist_bin8/7(Mxy_In11)
  [m_xy_21] -> hist_bin8/12(Mxy_In21)
  [orien_31] -> hist_bin8/42(Orien_In31)
  [orien_34] -> hist_bin8/45(Orien_In34)
  [m_xy_42] -> hist_bin8/23(Mxy_In42)
  [orien_01] -> hist_bin8/27(Orien_In01)
  [orien_00] -> hist_bin8/26(Orien_In00)
  [orien_04] -> hist_bin8/30(Orien_In04)
  [orien_13] -> hist_bin8/34(Orien_In13)
  [orien_20] -> hist_bin8/36(Orien_In20)
  [orien_24] -> hist_bin8/40(Orien_In24)
  [orien_33] -> hist_bin8/44(Orien_In33)
  [orien_32] -> hist_bin8/43(Orien_In32)
  [orien_41] -> hist_bin8/47(Orien_In41)
  [orien_11] -> hist_bin8/32(Orien_In11)
  [orien_21] -> hist_bin8/37(Orien_In21)
  [orien_14] -> hist_bin8/35(Orien_In14)
  [orien_22] -> hist_bin8/38(Orien_In22)
  [orien_23] -> hist_bin8/39(Orien_In23)
  [orien_02] -> hist_bin8/28(Orien_In02)
  [orien_10] -> hist_bin8/31(Orien_In10)
  [orien_12] -> hist_bin8/33(Orien_In12)
  [orien_30] -> hist_bin8/41(Orien_In30)
  [m_xy_44] -> hist_bin8/25(Mxy_In44)
  [orien_03] -> hist_bin8/29(Orien_In03)
  [orien_40] -> hist_bin8/46(Orien_In40)
  [clken] -> hist_bin8/51(clken)
  hist_bin8/1(bin_out) -> [hist_bin8]
  [orien_42] -> hist_bin8/48(Orien_In42)
  [orien_44] -> hist_bin8/50(Orien_In44)
  [orien_43] -> hist_bin8/49(Orien_In43)
  Constant7/1 -> hist_bin8/52(bin_in)
  [m_xy_00] -> hist_bin7/1(Mxy_In00)
  [hist_bin8] -> AltBus7/1
  [hist_bin7] -> AltBus6/1
  [hist_bin6] -> AltBus5/1
  [hist_bin5] -> AltBus4/1
  [hist_bin4] -> AltBus3/1
  [hist_bin3] -> AltBus2/1
  [hist_bin2] -> AltBus1/1
  [hist_bin1] -> AltBus/1
  [orien_22] -> Delay/1
  [clken] -> Delay/2
  Delay/1 -> AltBus8/1
  AltBus/1 -> Bus_Concatenation/2(bin1_in)
  AltBus1/1 -> Bus_Concatenation/3(bin2_in)
  AltBus2/1 -> Bus_Concatenation/4(biin3_in)
  AltBus3/1 -> Bus_Concatenation/5(bin4_in)
  AltBus4/1 -> Bus_Concatenation/6(bin5_in)
  AltBus5/1 -> Bus_Concatenation/7(bin6_in)
  AltBus6/1 -> Bus_Concatenation/8(bin_in)
  AltBus7/1 -> Bus_Concatenation/9(bin8_in)
  [clken] -> Bus_Concatenation/10(clken)
  Bus_Concatenation/1(hist_bin) -> hist_bin_out/1
  AltBus8/1 -> Bus_Concatenation/1(orien)
  Bus_Concatenation/2(Orien_out) -> Orien_out/1

== system SIFT_final/SIFT/SIFT_detector/Octave0 ==
  data_in : Inport
  valid_in : Inport  Port=2
  calculate_key_point : Subsystem
  dog_space : Subsystem
  scale_space : Subsystem
  Out1 : Outport
  scale2 : Outport  Port=2
  wires:
  scale_space/3(scale2) -> scale2/1, dog_space/3(scale2_in)
  scale_space/1(scale4) -> dog_space/1(scale4_in)
  scale_space/4(scale1) -> dog_space/4(scale1_in)
  calculate_key_point/1(is_KeyPoint) -> Out1/1
  scale_space/2(scale3) -> dog_space/2(scale3_in)
  dog_space/1(dog3_out) -> calculate_key_point/1(pixel_dog3_in)
  dog_space/3(dog1_out) -> calculate_key_point/3(pixel_dog1_in)
  dog_space/2(dog2_out) -> calculate_key_point/2(pixel_dog2_in)
  data_in/1 -> scale_space/1(data_in)
  valid_in/1 -> scale_space/2(valid_in), calculate_key_point/4(valid_in), dog_space/5(valid_in)

== system SIFT_final/SIFT/SIFT_detector/Octave1 ==
  data_in : Inport
  valid_in : Inport  Port=2
  Constant : allblocks_alteradspbuilder2/Constant  mask_cst=0  BusType=Unsigned Integer  bwl=1  bwr=0  roundMode=Truncate  satMode=Wrap  SpecifyClock=off  allowFloatingPointOverride=on  logOutputs=off  logFile=C:\Users\ASUS\Desktop\final_sift_fpga\tb_SIFT_final\SIFT%5Ffinal_SIFT_SIFT%5Fdetector_Octave1_Constant.fixedpointlog
  Multiplexer : allblocks_alteradspbuilder2/Multiplexer  numInputs=2  pipeline=0  oneHot=off  pipeline_display=0  use_ena=off  use_aclr=off  allowFloatingPointOverride=on  logOutputs=off  logFile=C:\Users\ASUS\Desktop\final_sift_fpga\tb_SIFT_final\SIFT%5Ffinal_SIFT_SIFT%5Fdetector_Octave1_Multiplexer.fixedpointlog
  calculate_key_point : Subsystem
  dog_space : Subsystem
  scale_space : Subsystem
  Out1 : Outport
  wires:
  scale_space/3(scale2) -> dog_space/3(scale2_in)
  scale_space/1(scale4) -> dog_space/1(scale4_in)
  scale_space/4(scale1) -> dog_space/4(scale1_in)
  calculate_key_point/1(is_KeyPoint) -> Multiplexer/3
  valid_in/1 -> scale_space/2(valid_in), Multiplexer/1, calculate_key_point/4(valid_in), dog_space/5(valid_in)
  scale_space/2(scale3) -> dog_space/2(scale3_in)
  dog_space/1(dog3_out) -> calculate_key_point/1(pixel_dog3_in)
  dog_space/3(dog1_out) -> calculate_key_point/3(pixel_dog1_in)
  dog_space/2(dog2_out) -> calculate_key_point/2(pixel_dog2_in)
  data_in/1 -> scale_space/1(data_in)
  Multiplexer/1 -> Out1/1
  Constant/1 -> Multiplexer/2

== system SIFT_final/SIFT/SIFT_detector/resize ==
  valid_in : Inport
  eof_in : Inport  Port=2
  sof_in : Inport  Port=3
  Comparator1 : allblocks_alteradspbuilder2/Comparator  direction=a == b  pipeline_display=0  allowFloatingPointOverride=on  logOutputs=off  logFile=C:\Users\ASUS\Desktop\final_sift_fpga\tb_SIFT_final\SIFT%5Ffinal_SIFT_SIFT%5Fdetector_resize_Comparator1.fixedpointlog
  Comparator2 : allblocks_alteradspbuilder2/Comparator  direction=a == b  pipeline_display=0  allowFloatingPointOverride=on  logOutputs=off  logFile=C:\Users\ASUS\Desktop\final_sift_fpga\tb_SIFT_final\SIFT%5Ffinal_SIFT_SIFT%5Fdetector_resize_Comparator2.fixedpointlog
  Comparator3 : allblocks_alteradspbuilder2/Comparator  direction=a == b  pipeline_display=0  allowFloatingPointOverride=on  logOutputs=off  logFile=C:\Users\ASUS\Desktop\final_sift_fpga\tb_SIFT_final\SIFT%5Ffinal_SIFT_SIFT%5Fdetector_resize_Comparator3.fixedpointlog
  Constant1 : allblocks_alteradspbuilder2/Constant  mask_cst=1  BusType=Unsigned Integer  bwl=2  bwr=0  roundMode=Truncate  satMode=Wrap  SpecifyClock=off  allowFloatingPointOverride=on  logOutputs=off  logFile=C:\Users\ASUS\Desktop\final_sift_fpga\tb_SIFT_final\SIFT%5Ffinal_SIFT_SIFT%5Fdetector_resize_Constant1.fixedpointlog
  Constant2 : allblocks_alteradspbuilder2/Constant  mask_cst=0  BusType=Unsigned Integer  bwl=2  bwr=0  roundMode=Truncate  satMode=Wrap  SpecifyClock=off  allowFloatingPointOverride=on  logOutputs=off  logFile=C:\Users\ASUS\Desktop\final_sift_fpga\tb_SIFT_final\SIFT%5Ffinal_SIFT_SIFT%5Fdetector_resize_Constant2.fixedpointlog
  Constant3 : allblocks_alteradspbuilder2/Constant  mask_cst=639  BusType=Unsigned Integer  bwl=10  bwr=0  roundMode=Truncate  satMode=Wrap  SpecifyClock=off  allowFloatingPointOverride=on  logOutputs=off  logFile=C:\Users\ASUS\Desktop\final_sift_fpga\tb_SIFT_final\SIFT%5Ffinal_SIFT_SIFT%5Fdetector_resize_Constant3.fixedpointlog
  Counter : allblocks_alteradspbuilder2/Counter  BusType=Unsigned Integer  bwl=2  bwr=0  use_modulo=on  modulo=2  SpecifyClock=off  direction=Increment  use_sload=off  use_sset=on  svalue=0  use_clk_ena=off  use_ena=on  use_sclr=on  pipeline_display=1
  Counter2 : allblocks_alteradspbuilder2/Counter  BusType=Unsigned Integer  bwl=10  bwr=0  use_modulo=on  modulo=640  SpecifyClock=off  direction=Increment  use_sload=off  use_sset=on  svalue=0  use_clk_ena=off  use_ena=on  use_sclr=on  pipeline_display=1
  Counter3 : allblocks_alteradspbuilder2/Counter  BusType=Unsigned Integer  bwl=2  bwr=0  use_modulo=on  modulo=2  SpecifyClock=off  direction=Increment  use_sload=off  use_sset=off  svalue=0  use_clk_ena=off  use_ena=on  use_sclr=on  pipeline_display=1
  Logical Bit Operator1 : allblocks_alteradspbuilder2/Logical Bit Operator  LogicalOperator=AND  user_inputs=3  pipeline_display=0
  Logical Bit Operator2 : allblocks_alteradspbuilder2/Logical Bit Operator  LogicalOperator=AND  user_inputs=2  pipeline_display=0
  select : Outport
  wires:
  eof_in/1 -> [eof_in]
  valid_in/1 -> [valid_in]
  Counter3/1 -> Comparator2/1
  Counter/1 -> Comparator1/1
  [valid_in] -> Counter/2
  sof_in/1 -> [sof_in]
  Constant1/1 -> Comparator1/2
  Comparator1/1 -> Logical Bit Operator1/1
  [eof_in] -> Counter/3
  Constant2/1 -> Comparator2/2
  Comparator2/1 -> Logical Bit Operator1/2
  Logical Bit Operator1/1 -> select/1
  [eof_in] -> Counter3/2
  Logical Bit Operator2/1 -> Counter3/1
  [counter_col] -> Comparator3/1
  Constant3/1 -> Comparator3/2
  Comparator3/1 -> Logical Bit Operator2/2
  Counter2/1 -> [counter_col]
  [valid_in] -> Counter2/2, Logical Bit Operator2/1
  [eof_in] -> Counter2/3
  [sof_in] -> Counter/1
  [sof_in] -> Counter2/1
  [valid_in] -> Logical Bit Operator1/3

== system SIFT_final/SIFT/Show_keypoint/show_key ==
  dataIn : Inport
  "is_keypoint " : Inport  Port=2
  clken : Inport  Port=3
  B : allblocks_alteradspbuilder2/Constant  mask_cst=39168  BusType=Unsigned Integer  bwl=24  bwr=0  roundMode=Truncate  satMode=Wrap  SpecifyClock=off  allowFloatingPointOverride=on  logOutputs=off  logFile=C:\Users\ASUS\Desktop\final_sift_fpga\tb_SIFT_final\SIFT%5Ffinal_SIFT_Show%5Fkeypoint_show%5Fkey_B.fixedpointlog
  B1 : allblocks_alteradspbuilder2/Constant  mask_cst=39168  BusType=Unsigned Integer  bwl=24  bwr=0  roundMode=Truncate  satMode=Wrap  SpecifyClock=off  allowFloatingPointOverride=on  logOutputs=off  logFile=C:\Users\ASUS\Desktop\final_sift_fpga\tb_SIFT_final\SIFT%5Ffinal_SIFT_Show%5Fkeypoint_show%5Fkey_B1.fixedpointlog
  B2 : allblocks_alteradspbuilder2/Constant  mask_cst=39168  BusType=Unsigned Integer  bwl=24  bwr=0  roundMode=Truncate  satMode=Wrap  SpecifyClock=off  allowFloatingPointOverride=on  logOutputs=off  logFile=C:\Users\ASUS\Desktop\final_sift_fpga\tb_SIFT_final\SIFT%5Ffinal_SIFT_Show%5Fkeypoint_show%5Fkey_B2.fixedpointlog
  G : allblocks_alteradspbuilder2/Constant  mask_cst=39168  BusType=Unsigned Integer  bwl=24  bwr=0  roundMode=Truncate  satMode=Wrap  SpecifyClock=off  allowFloatingPointOverride=on  logOutputs=off  logFile=C:\Users\ASUS\Desktop\final_sift_fpga\tb_SIFT_final\SIFT%5Ffinal_SIFT_Show%5Fkeypoint_show%5Fkey_G.fixedpointlog
  G1 : allblocks_alteradspbuilder2/Constant  mask_cst=39168  BusType=Unsigned Integer  bwl=24  bwr=0  roundMode=Truncate  satMode=Wrap  SpecifyClock=off  allowFloatingPointOverride=on  logOutputs=off  logFile=C:\Users\ASUS\Desktop\final_sift_fpga\tb_SIFT_final\SIFT%5Ffinal_SIFT_Show%5Fkeypoint_show%5Fkey_G1.fixedpointlog
  G2 : allblocks_alteradspbuilder2/Constant  mask_cst=39168  BusType=Unsigned Integer  bwl=24  bwr=0  roundMode=Truncate  satMode=Wrap  SpecifyClock=off  allowFloatingPointOverride=on  logOutputs=off  logFile=C:\Users\ASUS\Desktop\final_sift_fpga\tb_SIFT_final\SIFT%5Ffinal_SIFT_Show%5Fkeypoint_show%5Fkey_G2.fixedpointlog
  Memory Delay : allblocks_alteradspbuilder2/Memory Delay  BusType=Unsigned Integer  bwl=24  bwr=0  pipeline=637  pipeline_display=637  ram_type=AUTO  use_ena=on  use_sclr=off  allowFloatingPointOverride=on  logOutputs=off  logFile=C:\Users\ASUS\Desktop\final_sift_fpga\tb_SIFT_final\SIFT%5Ffinal_SIFT_Show%5Fkeypoint_show%5Fkey_Memory+Delay.fixedpointlog
  Memory Delay1 : allblocks_alteradspbuilder2/Memory Delay  BusType=Unsigned Integer  bwl=24  bwr=0  pipeline=637  pipeline_display=637  ram_type=AUTO  use_ena=on  use_sclr=off  allowFloatingPointOverride=on  logOutputs=off  logFile=C:\Users\ASUS\Desktop\final_sift_fpga\tb_SIFT_final\SIFT%5Ffinal_SIFT_Show%5Fkeypoint_show%5Fkey_Memory+Delay1.fixedpointlog
  Multiplexer : allblocks_alteradspbuilder2/Multiplexer  numInputs=2  pipeline=1  oneHot=off  pipeline_display=1  use_ena=on  use_aclr=off  allowFloatingPointOverride=on  logOutputs=off  logFile=C:\Users\ASUS\Desktop\final_sift_fpga\tb_SIFT_final\SIFT%5Ffinal_SIFT_Show%5Fkeypoint_show%5Fkey_Multiplexer.fixedpointlog
  Multiplexer1 : allblocks_alteradspbuilder2/Multiplexer  numInputs=2  pipeline=1  oneHot=off  pipeline_display=1  use_ena=on  use_aclr=off  allowFloatingPointOverride=on  logOutputs=off  logFile=C:\Users\ASUS\Desktop\final_sift_fpga\tb_SIFT_final\SIFT%5Ffinal_SIFT_Show%5Fkeypoint_show%5Fkey_Multiplexer1.fixedpointlog
  Multiplexer2 : allblocks_alteradspbuilder2/Multiplexer  numInputs=2  pipeline=1  oneHot=off  pipeline_display=1  use_ena=on  use_aclr=off  allowFloatingPointOverride=on  logOutputs=off  logFile=C:\Users\ASUS\Desktop\final_sift_fpga\tb_SIFT_final\SIFT%5Ffinal_SIFT_Show%5Fkeypoint_show%5Fkey_Multiplexer2.fixedpointlog
  Multiplexer3 : allblocks_alteradspbuilder2/Multiplexer  numInputs=2  pipeline=1  oneHot=off  pipeline_display=1  use_ena=on  use_aclr=off  allowFloatingPointOverride=on  logOutputs=off  logFile=C:\Users\ASUS\Desktop\final_sift_fpga\tb_SIFT_final\SIFT%5Ffinal_SIFT_Show%5Fkeypoint_show%5Fkey_Multiplexer3.fixedpointlog
  Multiplexer4 : allblocks_alteradspbuilder2/Multiplexer  numInputs=2  pipeline=1  oneHot=off  pipeline_display=1  use_ena=on  use_aclr=off  allowFloatingPointOverride=on  logOutputs=off  logFile=C:\Users\ASUS\Desktop\final_sift_fpga\tb_SIFT_final\SIFT%5Ffinal_SIFT_Show%5Fkeypoint_show%5Fkey_Multiplexer4.fixedpointlog
  Multiplexer5 : allblocks_alteradspbuilder2/Multiplexer  numInputs=2  pipeline=1  oneHot=off  pipeline_display=1  use_ena=on  use_aclr=off  allowFloatingPointOverride=on  logOutputs=off  logFile=C:\Users\ASUS\Desktop\final_sift_fpga\tb_SIFT_final\SIFT%5Ffinal_SIFT_Show%5Fkeypoint_show%5Fkey_Multiplexer5.fixedpointlog
  Multiplexer6 : allblocks_alteradspbuilder2/Multiplexer  numInputs=2  pipeline=1  oneHot=off  pipeline_display=1  use_ena=on  use_aclr=off  allowFloatingPointOverride=on  logOutputs=off  logFile=C:\Users\ASUS\Desktop\final_sift_fpga\tb_SIFT_final\SIFT%5Ffinal_SIFT_Show%5Fkeypoint_show%5Fkey_Multiplexer6.fixedpointlog
  Multiplexer7 : allblocks_alteradspbuilder2/Multiplexer  numInputs=2  pipeline=1  oneHot=off  pipeline_display=1  use_ena=on  use_aclr=off  allowFloatingPointOverride=on  logOutputs=off  logFile=C:\Users\ASUS\Desktop\final_sift_fpga\tb_SIFT_final\SIFT%5Ffinal_SIFT_Show%5Fkeypoint_show%5Fkey_Multiplexer7.fixedpointlog
  Multiplexer8 : allblocks_alteradspbuilder2/Multiplexer  numInputs=2  pipeline=1  oneHot=off  pipeline_display=1  use_ena=on  use_aclr=off  allowFloatingPointOverride=on  logOutputs=off  logFile=C:\Users\ASUS\Desktop\final_sift_fpga\tb_SIFT_final\SIFT%5Ffinal_SIFT_Show%5Fkeypoint_show%5Fkey_Multiplexer8.fixedpointlog
  RED : allblocks_alteradspbuilder2/Constant  mask_cst=39168  BusType=Unsigned Integer  bwl=24  bwr=0  roundMode=Truncate  satMode=Wrap  SpecifyClock=off  allowFloatingPointOverride=on  logOutputs=off  logFile=C:\Users\ASUS\Desktop\final_sift_fpga\tb_SIFT_final\SIFT%5Ffinal_SIFT_Show%5Fkeypoint_show%5Fkey_RED.fixedpointlog
  RED1 : allblocks_alteradspbuilder2/Constant  mask_cst=39168  BusType=Unsigned Integer  bwl=24  bwr=0  roundMode=Truncate  satMode=Wrap  SpecifyClock=off  allowFloatingPointOverride=on  logOutputs=off  logFile=C:\Users\ASUS\Desktop\final_sift_fpga\tb_SIFT_final\SIFT%5Ffinal_SIFT_Show%5Fkeypoint_show%5Fkey_RED1.fixedpointlog
  RED2 : allblocks_alteradspbuilder2/Constant  mask_cst=39168  BusType=Unsigned Integer  bwl=24  bwr=0  roundMode=Truncate  satMode=Wrap  SpecifyClock=off  allowFloatingPointOverride=on  logOutputs=off  logFile=C:\Users\ASUS\Desktop\final_sift_fpga\tb_SIFT_final\SIFT%5Ffinal_SIFT_Show%5Fkeypoint_show%5Fkey_RED2.fixedpointlog
  Out : Outport
  wires:
  dataIn/1 -> [data_in]
  [data_22] -> Out/1
  clken/1 -> [clken]
  "is_keypoint "/1 -> [is_keypoint]
  [data_in] -> Multiplexer/2
  [clken] -> Multiplexer/4
  [is_keypoint] -> Multiplexer/1
  RED/1 -> Multiplexer/3
  Multiplexer/1 -> Multiplexer1/2
  [clken] -> Multiplexer1/4
  [is_keypoint] -> Multiplexer1/1
  RED1/1 -> Multiplexer1/3
  Multiplexer1/1 -> Multiplexer2/2
  [clken] -> Multiplexer2/4
  [is_keypoint] -> Multiplexer2/1
  RED2/1 -> Multiplexer2/3
  Multiplexer2/1 -> Memory Delay/1
  [clken] -> Multiplexer3/4
  [is_keypoint] -> Multiplexer3/1
  B/1 -> Multiplexer3/3
  Multiplexer4/1 -> Multiplexer5/2
  [clken] -> Multiplexer5/4
  [is_keypoint] -> Multiplexer5/1
  B1/1 -> Multiplexer5/3
  Memory Delay1/1 -> Multiplexer6/2
  [clken] -> Multiplexer6/4
  [is_keypoint] -> Multiplexer6/1
  G/1 -> Multiplexer6/3
  Multiplexer6/1 -> Multiplexer7/2
  [clken] -> Multiplexer7/4
  [is_keypoint] -> Multiplexer7/1
  G1/1 -> Multiplexer7/3
  Multiplexer7/1 -> Multiplexer8/2
  [clken] -> Multiplexer8/4
  [is_keypoint] -> Multiplexer8/1
  G2/1 -> Multiplexer8/3
  [clken] -> Multiplexer4/4
  [is_keypoint] -> Multiplexer4/1
  B2/1 -> Multiplexer4/3
  Multiplexer3/1 -> Multiplexer4/2
  Multiplexer8/1 -> [data_22]
  [clken] -> Memory Delay/2
  Multiplexer5/1 -> Memory Delay1/1
  [clken] -> Memory Delay1/2
  Memory Delay/1 -> Multiplexer3/2

== system SIFT_final/SIFT/Calculate_descriptor/GradOrien/lineBuff_3x3 ==
  dataIn : Inport
  clken : Inport  Port=2
  Delay : allblocks_alteradspbuilder2/Delay  pipeline=1  pipeline_display=1  ClockPhase=1  use_ena=on  use_sclr=off  allowFloatingPointOverride=on  logOutputs=off  logFile=C:\Users\ASUS\Desktop\final_sift_fpga\tb_SIFT_detection_feature\SIFT%5Fdetection%5Ffeature_calculate%5Fdescriptor_GradOrien_lineBuff%5F3x3_Delay.fixedpointlog  use_init=off  reset_value=1
  Delay1 : allblocks_alteradspbuilder2/Delay  pipeline=1  pipeline_display=1  ClockPhase=1  use_ena=on  use_sclr=off  allowFloatingPointOverride=on  logOutputs=off  logFile=C:\Users\ASUS\Desktop\final_sift_fpga\tb_SIFT_detection_feature\SIFT%5Fdetection%5Ffeature_calculate%5Fdescriptor_GradOrien_lineBuff%5F3x3_Delay1.fixedpointlog  use_init=off  reset_value=1
  Delay2 : allblocks_alteradspbuilder2/Delay  pipeline=1  pipeline_display=1  ClockPhase=1  use_ena=on  use_sclr=off  allowFloatingPointOverride=on  logOutputs=off  logFile=C:\Users\ASUS\Desktop\final_sift_fpga\tb_SIFT_detection_feature\SIFT%5Fdetection%5Ffeature_calculate%5Fdescriptor_GradOrien_lineBuff%5F3x3_Delay2.fixedpointlog  use_init=off  reset_value=1
  Delay5 : allblocks_alteradspbuilder2/Delay  pipeline=1  pipeline_display=1  ClockPhase=1  use_ena=on  use_sclr=off  allowFloatingPointOverride=on  logOutputs=off  logFile=C:\Users\ASUS\Desktop\final_sift_fpga\tb_SIFT_detection_feature\SIFT%5Fdetection%5Ffeature_calculate%5Fdescriptor_GradOrien_lineBuff%5F3x3_Delay5.fixedpointlog  use_init=off  reset_value=1
  Delay6 : allblocks_alteradspbuilder2/Delay  pipeline=1  pipeline_display=1  ClockPhase=1  use_ena=on  use_sclr=off  allowFloatingPointOverride=on  logOutputs=off  logFile=C:\Users\ASUS\Desktop\final_sift_fpga\tb_SIFT_detection_feature\SIFT%5Fdetection%5Ffeature_calculate%5Fdescriptor_GradOrien_lineBuff%5F3x3_Delay6.fixedpointlog  use_init=off  reset_value=1
  Delay9 : allblocks_alteradspbuilder2/Delay  pipeline=1  pipeline_display=1  ClockPhase=1  use_ena=on  use_sclr=off  allowFloatingPointOverride=on  logOutputs=off  logFile=C:\Users\ASUS\Desktop\final_sift_fpga\tb_SIFT_detection_feature\SIFT%5Fdetection%5Ffeature_calculate%5Fdescriptor_GradOrien_lineBuff%5F3x3_Delay9.fixedpointlog  use_init=off  reset_value=1
  Memory Delay : allblocks_alteradspbuilder2/Memory Delay  BusType=Inferred  bwl=9  bwr=16  pipeline=638  pipeline_display=638  ram_type=AUTO  use_ena=on  use_sclr=off  allowFloatingPointOverride=on  logOutputs=off  logFile=C:\Users\ASUS\Desktop\final_sift_fpga\tb_SIFT_detection_feature\SIFT%5Fdetection%5Ffeature_calculate%5Fdescriptor_GradOrien_lineBuff%5F3x3_Memory+Delay.fixedpointlog
  Memory Delay1 : allblocks_alteradspbuilder2/Memory Delay  BusType=Inferred  bwl=9  bwr=16  pipeline=638  pipeline_display=638  ram_type=AUTO  use_ena=on  use_sclr=off  allowFloatingPointOverride=on  logOutputs=off  logFile=C:\Users\ASUS\Desktop\final_sift_fpga\tb_SIFT_detection_feature\SIFT%5Fdetection%5Ffeature_calculate%5Fdescriptor_GradOrien_lineBuff%5F3x3_Memory+Delay1.fixedpointlog
  Out01 : Outport
  Out10 : Outport  Port=2
  Out12 : Outport  Port=3
  Out21 : Outport  Port=4
  wires:
  Delay1/1 -> [data_01], Delay2/1
  [clken] -> Memory Delay1/2
  Delay6/1 -> Memory Delay1/1, [data_12]
  Memory Delay1/1 -> Delay9/1
  [clken] -> Delay9/2
  [clken] -> Delay1/2
  [clken] -> Delay/2
  [data_in] -> Delay/1
  [clken] -> Delay2/2
  Delay2/1 -> Memory Delay/1
  clken/1 -> [clken]
  [data_21] -> Out21/1
  [data_10] -> Out10/1
  Memory Delay/1 -> [data_10], Delay5/1
  [clken] -> Memory Delay/2
  [clken] -> Delay6/2
  Delay5/1 -> Delay6/1
  [data_12] -> Out12/1
  [data_01] -> Out01/1
  [clken] -> Delay5/2
  dataIn/1 -> [data_in]
  Delay9/1 -> [data_21]
  Delay/1 -> Delay1/1
